simulink model "Eva_Buenafe_O_SIMULINK_1"  (R2023b)
settings: Solver=VariableStepAuto  StartTime=0.0  StopTime=20.0  RelTol=1e-3
values from neighbouring files (symbols this model uses):
  G_den = [b c d]    [Buenafe_Eva_O_MATLAB_1.m]    (also in Buenafe_Eva_O_MATLAB_2.m; Ebora_Zandro_Zevastien_Zyn_A_MATLAB_5_and_6.m = [1 2 3 4 1]; Rago_MATLAB_No3.m; Rago_MATLAB_No4.m = [b c])
  G_num = [a]    [Buenafe_Eva_O_MATLAB_1.m]    (also in Buenafe_Eva_O_MATLAB_2.m; Ebora_Zandro_Zevastien_Zyn_A_MATLAB_5_and_6.m = [4 3 2 1]; Rago_MATLAB_No3.m; Rago_MATLAB_No4.m)
settings Model: Creator=Ralph Rago  LastModifiedBy=Ralph Rago

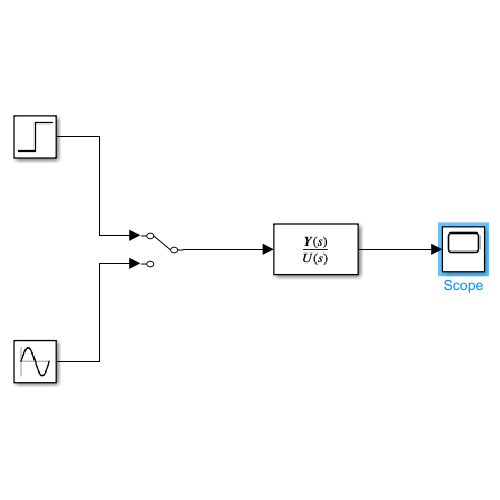
[thumbnail: Simulink's stored preview of the top-level diagram]
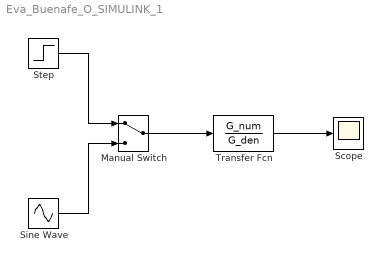
== system Eva_Buenafe_O_SIMULINK_1 ==
  Manual Switch : ManualSwitch
  Scope : Scope
  Sine Wave : Sin  SampleTime=0
  Step : Step  Time=0.1  SampleTime=0
  Transfer Fcn : TransferFcn  Numerator=G_num  Denominator=G_den
  wires:
  Sine Wave/1 -> Manual Switch/2
  Manual Switch/1 -> Transfer Fcn/1
  Step/1 -> Manual Switch/1
  Transfer Fcn/1 -> Scope/1
